simulink library "LaneDetection"  (R2024b)
settings: Solver=VariableStepAuto  StartTime=0.0  StopTime=10.0  RelTol=1e-3
values from neighbouring files (symbols this model uses):
  LaneWidth = 3.85    [RRStartUp.m]    (also in StartUp.m)
settings Model: Creator=austi  LastModifiedBy=wshei

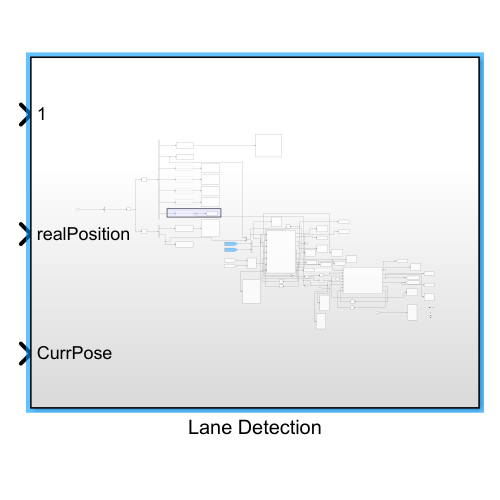
[thumbnail: Simulink's stored preview of the top-level diagram]
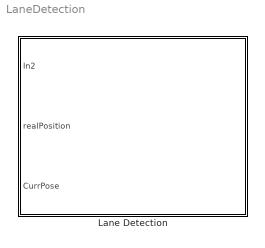
== system LaneDetection ==
  Lane Detection : Subsystem

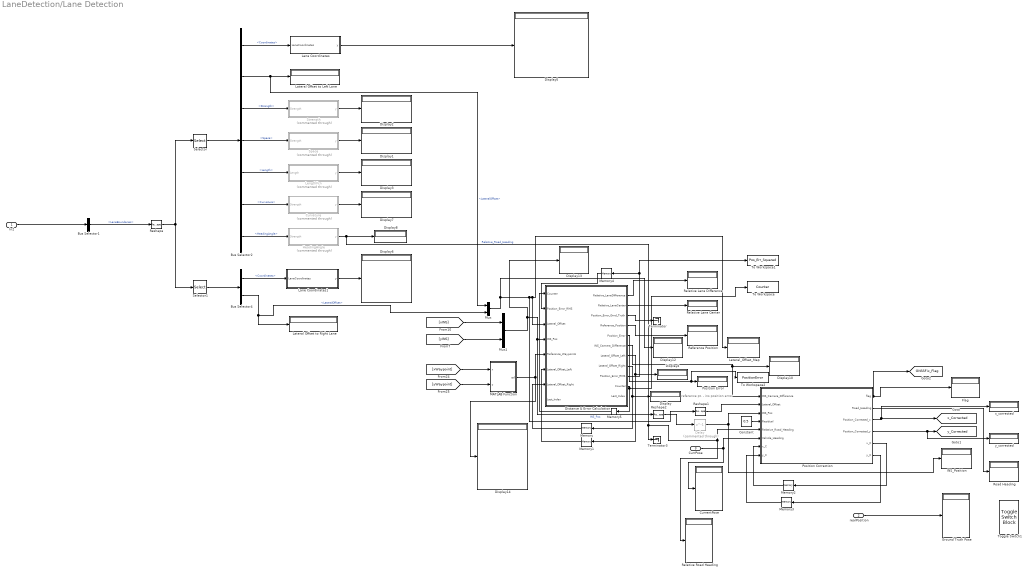
== system LaneDetection/Lane Detection ==
  note: reference pt. - ins position error
  In2 : Inport
  realPosition : Inport  Port=2
  CurrPose : Inport  Port=3
  Bus Selector1 : BusSelector  OutputSignals=LaneBoundaries
  Bus Selector2 : BusSelector  OutputSignals=Coordinates,LateralOffset,Strength,Space,Length,Curvature,HeadingAngle
  Bus Selector4 : BusSelector  OutputSignals=Coordinates,LateralOffset
  Constant : Constant  Value=0.5
  CurrentPose : Display
  Curvature : MATLAB Function  Commented=through  TreatAsAtomicUnit=on
  Delay : Delay  Commented=through  DelayLength=1
  Display{,1..8,10,12..14} (13 alike) : Display
  Distance & Error Calculation : MATLAB Function  TreatAsAtomicUnit=on
  Flag : Display
  Ground Truth Pose : Display
  HeadingAngle : MATLAB Function  Commented=through  TreatAsAtomicUnit=on
  INS_Position : Display
  Lane Coordinates : MATLAB Function  TreatAsAtomicUnit=on
  Lane Coordinates1 : MATLAB Function  TreatAsAtomicUnit=on
  Lateral Offset to Left Lane : Display
  Lateral Offset to Right Lane : Display
  Lateral_Offset_Map : Display
  LengthFcn : MATLAB Function  Commented=through  TreatAsAtomicUnit=on
  MATLAB Function : MATLAB Function  TreatAsAtomicUnit=on
  Memory : Memory  InitialCondition=LaneWidth/2
  Memory1 : Memory  InitialCondition=LaneWidth/2
  Memory{2..5} (4 alike) : Memory
  Mux : Mux  Inputs=2
  Mux1 : Mux  Inputs=2
  Position Correction : MATLAB Function  TreatAsAtomicUnit=on
  Position Error : Display
  Reference Position : Display
  Relative Lane Center : Display
  Relative Lane Difference : Display
  Relative Road Heading : Display
  Reshape : Reshape  OutputDimensionality=Customize  OutputDimensions=[500, 1]
  Reshape1 : Reshape  OutputDimensionality=Column vector (2-D)
  Reshape2 : Reshape  OutputDimensionality=Column vector (2-D)
  Road Heading : Display
  Selector : Selector  InputPortWidth=500  IndexOptions=Index vector (dialog)  Indices=[1]  OutputSizes=1
  Selector1 : Selector  InputPortWidth=500  IndexOptions=Index vector (dialog)  Indices=[2]  OutputSizes=1
  Space : MATLAB Function  Commented=through  TreatAsAtomicUnit=on
  Strength : MATLAB Function  Commented=through  TreatAsAtomicUnit=on
  Terminator : Terminator
  Terminator3 : Terminator
  To Workspace : ToWorkspace  VariableName=Counter  SaveFormat=Structure  SampleTime=-1
      settings: Save2DSignal=2-D array (concatenate along first dimension)
  To Workspace1 : ToWorkspace  VariableName=Pos_Err_Squared  SaveFormat=Structure  SampleTime=-1
      settings: Save2DSignal=2-D array (concatenate along first dimension)
  To Workspace2 : ToWorkspace  VariableName=PositionError  SaveFormat=Timeseries  SampleTime=-1
  Toggle Switch1 : ToggleSwitchBlock
      settings: Values={{'Off', 'On'}, [0 1]}
  x_corrected : Display
  y_corrected : Display
  tag scope: GNSSFix_Flag=global, x_Corrected=global, y_Corrected=global
  wires:
  Lane Coordinates/1(y) -> Display5/1
  Bus Selector4/1 -> Lane Coordinates1/1(LaneCoordinates)  "<Coordinates>"
  Lane Coordinates1/1(y) -> Display6/1
  In2/1 -> Bus Selector1/1
  Selector1/1 -> Bus Selector4/1
  Reshape/1 -> Selector/1, Selector1/1
  Bus Selector2/1 -> Lane Coordinates/1(LaneCoordinates)  "<Coordinates>"
  Selector/1 -> Bus Selector2/1
  Bus Selector1/1 -> Reshape/1  "<LaneBoundaries>"
  Bus Selector2/2 -> Mux/1, Lateral Offset to Left Lane/1  "<LateralOffset>"
  Bus Selector2/3 -> Strength/1(Strength)  "<Strength>"
  Bus Selector2/4 -> Space/1(Strength)  "<Space>"
  Bus Selector2/5 -> LengthFcn/1(Length)  "<Length>"
  Bus Selector2/6 -> Curvature/1(Strength)  "<Curvature>"
  Curvature/1(y) -> Display7/1
  Bus Selector2/7 -> HeadingAngle/1(Strength)  "<HeadingAngle>"
  Bus Selector4/2 -> Mux/2, Lateral Offset to Right Lane/1  "<LateralOffset>"
  Space/1(y) -> Display1/1
  Strength/1(y) -> Display2/1
  LengthFcn/1(y) -> Display3/1
  Mux1/1 -> Display13/1, Reshape2/1, Distance & Error Calculation/4(INS_Pos)  "INS_Pos"
  [xINS] -> Mux1/1
  [yINS] -> Mux1/2
  [xWaypoint] -> MATLAB Function/1(x)
  [yWaypoint] -> MATLAB Function/2(y)
  MATLAB Function/1(ref) -> Distance & Error Calculation/5(Reference_Waypoints), Display14/1
  Distance & Error Calculation/1(Relative_LaneDifference) -> Relative Lane Difference/1
  Distance & Error Calculation/6(INS_Camera_Difference) -> Position Correction/1(INS_Camera_Difference), Display10/1
  Distance & Error Calculation/4(Reference_Position) -> Reference Position/1
  Distance & Error Calculation/5(Position_Error) -> To Workspace2/1, Position Error/1
  Mux/1 -> Display12/1, Reshape1/1, Lateral_Offset_Map/1, Distance & Error Calculation/3(Lateral_Offset)
  Distance & Error Calculation/2(Relative_LaneCenter) -> Relative Lane Center/1
  Distance & Error Calculation/3(Position_Error_Grnd_Truth) -> Terminator/1
  Distance & Error Calculation/7(Lateral_Offset_Left) -> Memory1/1, Display4/1
  Distance & Error Calculation/8(Lateral_Offset_Right) -> Display/1, Memory/1
  Memory/1 -> Distance & Error Calculation/7("Lateral_Offset_Right ")
  Memory1/1 -> Distance & Error Calculation/6("Lateral_Offset_Left ")
  Constant/1 -> Position Correction/4(Residual)
  CurrPose/1 -> CurrentPose/1, Position Correction/6(Vehicle_Heading)
  Reshape1/1 -> Position Correction/2(Lateral_Offset)
  Reshape2/1 -> Delay/1
  Position Correction/6(y_C) -> Memory3/1
  HeadingAngle/1(y) -> Position Correction/5(Relative_Road_Heading), Relative Road Heading/1, Terminator3/1, Display8/1  "Relative_Road_Heading"
  Position Correction/5(x_C) -> Memory2/1
  Position Correction/2(Road_Heading) -> Road Heading/1
  realPosition/1 -> Ground Truth Pose/1
  Memory2/1 -> Position Correction/7("x_C ")
  Memory3/1 -> Position Correction/8("y_C ")
  Position Correction/3(Position_Corrected_x) -> [x_Corrected], x_corrected/1
  Position Correction/4(Position_Corrected_y) -> y_corrected/1, [y_Corrected]
  Delay/1 -> Position Correction/3(INS_Pos), INS_Position/1
  Position Correction/1(flag) -> [GNSSFix_Flag], Flag/1
  Distance & Error Calculation/9(Position_Error_RMS) -> To Workspace1/1, Memory4/1
  Memory4/1 -> Distance & Error Calculation/2("Position_Error_RMS ")
  Distance & Error Calculation/10(Counter) -> Memory5/1, To Workspace/1
  Memory5/1 -> Distance & Error Calculation/1("Counter ")

== matlab function LaneDetection/Lane Detection/LengthFcn ==
  data: Length input; y output
function y = fcn(Length)

y = Length(1:20, 1:3);

== matlab function LaneDetection/Lane Detection/Space ==
  data: Strength input; y output
function y = fcn(Strength)

y = Strength(1:20, 1:3);

== matlab function LaneDetection/Lane Detection/Curvature ==
  data: Strength input; y output
function y = fcn(Strength)

y = Strength(1:20, 1:3);

== matlab function LaneDetection/Lane Detection/HeadingAngle ==
  data: Strength input; y output
function y = fcn(Strength)

y = Strength(1:20, 1:3);

== matlab function LaneDetection/Lane Detection/Distance & Error Calculation ==
  data: Counter input; Position_Error_RMS input; Lateral_Offset input; Relative_LaneDifference output; Relative_LaneCenter output; Position_Error_Grnd_Truth output; INS_Pos input; Reference_Waypoints input; Reference_Position output; Position_Error output; INS_Camera_Difference output; Lateral_Offset_Left input; Lateral_Offset_Right input; Lateral_Offset_Left output; Lateral_Offset_Right output; Position_Error_RMS output; Counter output; Last_Index input; Last_Index output
function [Relative_LaneDifference, Relative_LaneCenter, Position_Error_Grnd_Truth, Reference_Position, Position_Error, INS_Camera_Difference, Lateral_Offset_Left, Lateral_Offset_Right, Position_Error_RMS, Counter, Last_Index] ...
    = DistanceCalculation(Counter, Position_Error_RMS, Lateral_Offset, INS_Pos, Reference_Waypoints, Lateral_Offset_Left, Lateral_Offset_Right, Last_Index)

    % --- 1. MANDATORY INITIALIZATION ---
    % Pre-defining these ensures Simulink always knows the size of your outputs
    Reference_Position = zeros(1, 2);
    Relative_LaneDifference = zeros(1, 2);
    INS_Camera_Difference = zeros(1, 2);
    INS_Location = [INS_Pos(1), INS_Pos(2)];
    
    Position_Error = 0;
    Position_Error_Grnd_Truth = 0;
    Relative_LaneCenter = 0;

    % --- 2. TRAJECTORY LOCKING LOGIC ---
    Num_Waypoints = size(Reference_Waypoints, 1);
    
    % Use a persistent index to "lock" the car to a specific lane trajectory
    if Counter <= 1 || Last_Index <= 0
        Dist_Sq = sum((Reference_Waypoints(:, 1:2) - INS_Location).^2, 2);
        [~, min_idx] = min(Dist_Sq);
        Last_Index = min_idx;
    end
    
    % Search window of +/- 10 indices around the last known position
    Window_Size = 10;
    Start_Idx = max(1, floor(Last_Index) - Window_Size);
    End_Idx = min(Num_Waypoints, floor(Last_Index) + Window_Size);
    Search_Range = Start_Idx:End_Idx;
    
    % Local search prevents jumping to adjacent lanes
    Window_Points = Reference_Waypoints(Search_Range, 1:2);
    Window_Dists = sum((Window_Points - INS_Location).^2, 2);
    [~, local_min] = min(Window_Dists);
    
    % Update the index for the next step
    Last_Index = double(Search_Range(local_min)); 
    
    % Define the segment for interpolation
    if Last_Index < Num_Waypoints
        idx1 = int32(Last_Index);
        idx2 = int32(Last_Index + 1);
    else
        idx1 = int32(Last_Index - 1);
        idx2 = int32(Last_Index);
    end
    
    % --- 3. POSITION CALCULATION ---
    P1 = Reference_Waypoints(idx1, 1:2);
    P2 = Reference_Waypoints(idx2, 1:2);
    DX = P2(1) - P1(1);
    DY = P2(2) - P1(2);
    
    if abs(DX) < 1e-6 
        Reference_Position = [P1(1), INS_Location(2)];
    elseif abs(DY) < 1e-6 
        Reference_Position = [INS_Location(1), P1(2)];
    else
        Slope = DY / DX;
        Intercept1 = P1(2) - Slope * P1(1);
        OrthSlope = -1/Slope;
        Intercept2 = INS_Location(2) - OrthSlope * INS_Location(1);
        RefX = (Intercept2 - Intercept1) / (Slope - OrthSlope);
        RefY = Slope * RefX + Intercept1;
        Reference_Position = [RefX, RefY];
    end
    
    % --- 4. STATISTICS & ERRORS ---
    Position_Error = sqrt(sum((Reference_Position - INS_Location).^2));
    Position_Error_RMS = Position_Error_RMS + (Position_Error^2);
    Counter = Counter + 1;
    Position_Error_Grnd_Truth = Position_Error; 
    
    % --- 5. LANE OFFSET LOGIC ---
    if (Lateral_Offset(1) < 5 && Lateral_Offset(1) > 0) && (Lateral_Offset(2) > -5 && Lateral_Offset(2) < 0)
        L_Lat = Lateral_Offset(1);
        R_Lat = abs(Lateral_Offset(2));
    else
        L_Lat = 1.6925; 
        R_Lat = 1.6925;
    end
    
    Lateral_Offset_Left = L_Lat;
    Lateral_Offset_Right = R_Lat;
    Relative_LaneCenter = (L_Lat + R_Lat) / 2;
    Relative_LaneDifference = [abs(L_Lat - Relative_LaneCenter), abs(R_Lat - Relative_LaneCenter)];
    
    INS_Camera_Difference(1) = Relative_LaneDifference(1) - Position_Error;
    INS_Camera_Difference(2) = Relative_LaneDifference(2) - Position_Error;
end
    
    %{
    Relative_LaneCenter = 0;
    Distance2Ref = zeros(length(Reference_Waypoints), 1);
    
    Position_Error = 0;
    Position_Error_Grnd_Truth = 0;
    
    
    % Change based on distance between two points
    for i = 1: length(Reference_Waypoints)
        Distance2Ref(i) = norm(INS_Location(1:2) - Reference_Waypoints(i, 1:2));
    end

    [~, index] = mink(Distance2Ref, 2);

    if index(1) > index(2)
        index = [index(2); index(1)];
    end

    % INS_Position & Reference Position Error
    Slope = 0; Orth_Slope = 0; C_Intercept_1 = 0; C_Intercept_2 = 0;

    Slope = (Reference_Waypoints(index(1), 2) - Reference_Waypoints(index(2), 2)) / (Reference_Waypoints(index(1), 1) - Reference_Waypoints(index(2), 1));

    if Slope >= 1e4
        Reference_Position = [Reference_Waypoints(index(1), 1), INS_Location(2)];
    elseif Slope <= 1e-4
        Reference_Position = [INS_Location(1), Reference_Waypoints(index(1), 2)];
    else
        C_Intercept_1 = Reference_Waypoints(index(1), 2) - Slope*Reference_Waypoints(index(1), 1);
        Orth_Slope = -1/Slope;
        C_Intercept_2 = INS_Location(2) - Orth_Slope*INS_Location(1);
        Reference_Position(1:2) = [(C_Intercept_1 - C_Intercept_2) / (Orth_Slope - Slope), Slope*(C_Intercept_1 - C_Intercept_2) / ((Orth_Slope - Slope)) + C_Intercept_1];
    end

    Position_Error = norm(Reference_Position(1:2) - INS_Location(1:2));
    Position_Error_RMS = Position_Error_RMS + Position_Error^2;
    Counter = Counter + 1;
    

    % Position_Error_Grnd_Truth = norm(Reference_Position(:, 1:2) - Real_Position(1:2));
    
    if (Lateral_Offset(1) < 5 && Lateral_Offset(1) > 0) && (Lateral_Offset(2) > -5 && Lateral_Offset(2) < 0)
        LateralOffset_LeftLane = Lateral_Offset(1);
        LateralOffset_RightLane = abs(Lateral_Offset(2));

        Lateral_Offset_Left = LateralOffset_LeftLane;
        Lateral_Offset_Right = LateralOffset_RightLane;
    else
        LateralOffset_LeftLane = 6.77/2/2;
        LateralOffset_RightLane = 6.77/2/2;

        Lateral_Offset_Left = LateralOffset_LeftLane;
        Lateral_Offset_Right = LateralOffset_RightLane;
    end

    % Camera Offset / Difference Calculation
    Relative_LaneCenter = (Lateral_Offset_Left + Lateral_Offset_Right) / 2;
    Relative_LaneDifference = [abs(LateralOffset_LeftLane - Relative_LaneCenter), abs(LateralOffset_RightLane - Relative_LaneCenter)];

    % INS Position - Camera Position Difference
    INS_Camera_Difference(1) = Relative_LaneDifference(1) - Position_Error;
    INS_Camera_Difference(2) = Relative_LaneDifference(2) - Position_Error;
    
end
    %}

== matlab function LaneDetection/Lane Detection/Lane Coordinates ==
  data: LaneCoordinates input; y output
function y  = fcn(LaneCoordinates)

y = LaneCoordinates(1:20, 1:3);
y2 = LaneCoordinates(1, 2);

end

== matlab function LaneDetection/Lane Detection/Lane Coordinates1 ==
  data: LaneCoordinates input; y output
function y = fcn(LaneCoordinates)

y = LaneCoordinates(1:10, 1:2);

== matlab function LaneDetection/Lane Detection/MATLAB Function ==
  data: x input; ref output; y input
function ref = fcn(x, y)

    ref = [x, y];
end

== matlab function LaneDetection/Lane Detection/Position Correction ==
  data: flag output; Road_Heading output; INS_Camera_Difference input; Lateral_Offset input; INS_Pos input; Residual input; Relative_Road_Heading input; Vehicle_Heading input; Position_Corrected_x output; Position_Corrected_y output; x_C input; y_C input; x_C output; y_C output
function [flag, Road_Heading, Position_Corrected_x, Position_Corrected_y, x_C, y_C]  = ResidualCalculation(INS_Camera_Difference, Lateral_Offset, INS_Pos, Residual, Relative_Road_Heading, Vehicle_Heading, x_C, y_C)
    
    Road_Heading = Vehicle_Heading(3) + Relative_Road_Heading(1);
    % flag = zeros(1, 1);
    

    Position_Corrected_x = 0;
    Position_Corrected_y = 0;

    if (Lateral_Offset(1) < 5 && Lateral_Offset(1) > 0) && (Lateral_Offset(2) > -5 && Lateral_Offset(2) < 0) && (abs(INS_Camera_Difference(1)) >= Residual)
         flag = ones(1, 1);
         x1 = sind(Road_Heading);
         x2 = cosd(Road_Heading);
         
         Position_Corrected_x = INS_Pos(1) - (INS_Camera_Difference(1) * x2);
         Position_Corrected_y = INS_Pos(2) + (INS_Camera_Difference(1) * x1);
         % Heading_Corrected = 
         x_C = Position_Corrected_x;
         y_C = Position_Corrected_y;
    else
        flag = zeros(1, 1);
        if x_C == 0 && y_C == 0
            Position_Corrected_x = INS_Pos(1);
            Position_Corrected_y = INS_Pos(2);
        else
            Position_Corrected_x = x_C;
            Position_Corrected_y = y_C;
        end
    end

== matlab function LaneDetection/Lane Detection/Strength ==
  data: Strength input; y output
function y = fcn(Strength)

y = Strength(1:20, 1:3);
